simulink model "sim_continuo_vs_discreto_control_integral"  (R2016a)
settings: Solver=VariableStepAuto  StartTime=0.0  StopTime=0.2  RelTol=1e-5
values from neighbouring files (symbols this model uses):
  A = [0 1 ... (first row only)    [calculate_gains.m]    (also in get_linear_model.m = jacobian(xp_nl,x_state))
  B = [0 ... (first row only)    [calculate_gains.m]    (also in get_linear_model.m = jacobian(xp_nl,u_state))
  C = [1 0]    [calculate_gains.m]    (also in get_linear_model.m = jacobian(y_nl,x_state))
  Kdi = calc_discrete_integral_controller_gains(A,B,C,Pi,Ts)    [generate_lookup_table.m]
  Ki = calc_integral_controller_gains(A,B,C,Pi)    [generate_lookup_table.m]
  Ts = 4e-4    (= 0.0004)    [calculate_gains.m]    (also in generate_lookup_table.m = 0.0005)
undefined symbols (not defined in the file or in its folder): Ad, Bd, Cd, DiscIntNeverNeededParam, Kdo, Ko
settings Model: Creator=manuel  LastModifiedBy=manuel

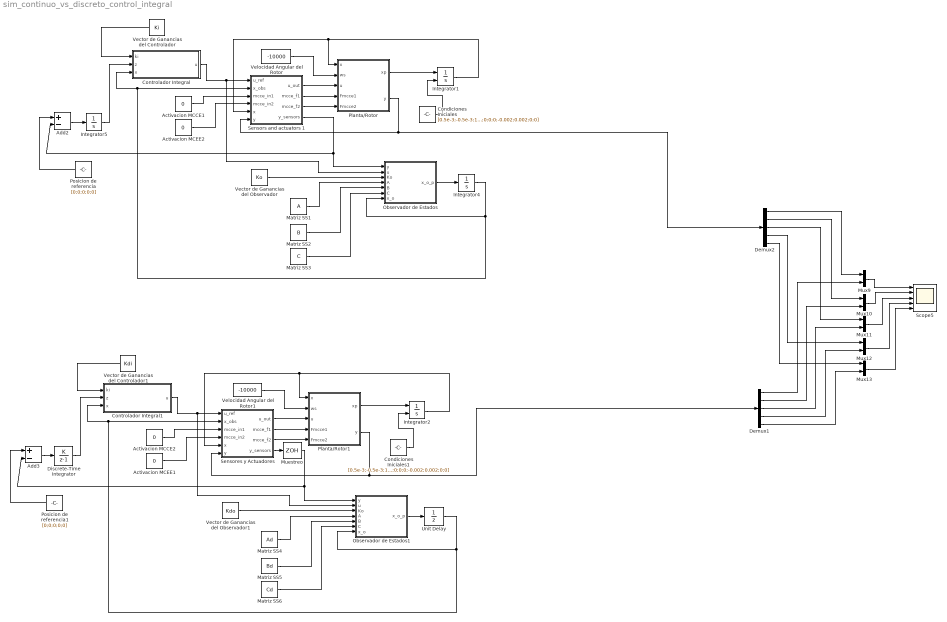
== system sim_continuo_vs_discreto_control_integral ==
  Activacion MCCE1 : Constant  Value=0
  Activacion MCCE2 : Constant  Value=0
  Activacion MCEE1 : Constant  Value=0
  Activacion MCEE2 : Constant  Value=0
  Add2 : Sum  Inputs=+-
  Add3 : Sum  Inputs=+-
  Condiciones Iniciales : Constant  Value=[0.5e-3;-0.5e-3;1e-3;0;0;0;-0.002;0.002;0;0]
  Condiciones Iniciales1 : Constant  Value=[0.5e-3;-0.5e-3;1e-3;0;0;0;-0.002;0.002;0;0]
  Controlador Integral : MATLAB Function  TreatAsAtomicUnit=on
  Controlador Integral1 : MATLAB Function  TreatAsAtomicUnit=on
  Demux1 : Demux  Outputs=5
  Demux2 : Demux  Outputs=5
  Discrete-Time Integrator : DiscreteIntegrator  IntegratorMethod=Accumulation: Forward Euler  gainval=1  InitialCondition=[0;0;0;0;0]  InitialConditionSetting=State (most efficient)  SampleTime=-1  ICPrevOutput=DiscIntNeverNeededParam  ICPrevScaledInput=DiscIntNeverNeededParam
  Integrator1 : Integrator  InitialConditionSource=external  InitialCondition=[0;0;0;0;0;0;0;0;0;0]
  Integrator2 : Integrator  InitialConditionSource=external  InitialCondition=[0;0;0;0;0;0;0;0;0;0]
  Integrator4 : Integrator  InitialCondition=[0;0;0;0;0;0;0;0;0;0]
  Integrator5 : Integrator  InitialCondition=[0;0;0;0;0]
  Matriz SS1 : Constant  Value=A  VectorParams1D=off
  Matriz SS2 : Constant  Value=B  VectorParams1D=off
  Matriz SS3 : Constant  Value=C  VectorParams1D=off
  Matriz SS4 : Constant  Value=Ad  VectorParams1D=off
  Matriz SS5 : Constant  Value=Bd  VectorParams1D=off
  Matriz SS6 : Constant  Value=Cd  VectorParams1D=off
  Muestreo : ZeroOrderHold  SampleTime=Ts
  Mux{9..13} (5 alike) : Mux  Inputs=2
  Observador de Estados : MATLAB Function  TreatAsAtomicUnit=on
  Observador de Estados1 : MATLAB Function  TreatAsAtomicUnit=on
  Planta/Rotor : MATLAB Function  TreatAsAtomicUnit=on
  Planta/Rotor1 : MATLAB Function  TreatAsAtomicUnit=on
  Posicion de referencia : Constant  Value=[0;0;0;0;0]
  Posicion de referencia1 : Constant  Value=[0;0;0;0;0]
  Scope5 : Scope  NumInputPorts=5
  Sensores y Actuadores : Subsystem
  Sensors and actuators 1 : Subsystem
  Unit Delay : UnitDelay  InitialCondition=[0;0;0;0;0;0;0;0;0;0]  SampleTime=-1
  Vector de Ganancias del Controlador : Constant  Value=Ki  VectorParams1D=off
  Vector de Ganancias del Controlador1 : Constant  Value=Kdi  VectorParams1D=off
  Vector de Ganancias del Observador : Constant  Value=Ko  VectorParams1D=off
  Vector de Ganancias del Observador1 : Constant  Value=Kdo  VectorParams1D=off
  Velocidad Angular del Rotor : Constant  Value=-10000  VectorParams1D=off
  Velocidad Angular del Rotor1 : Constant  Value=-10000  VectorParams1D=off
  wires:
  Mux9/1 -> Scope5/1
  Mux10/1 -> Scope5/2
  Mux11/1 -> Scope5/3
  Mux12/1 -> Scope5/4
  Mux13/1 -> Scope5/5
  Demux1/2 -> Mux10/2
  Demux1/1 -> Mux9/2
  Demux1/3 -> Mux11/2
  Demux1/4 -> Mux12/2
  Demux1/5 -> Mux13/2
  Demux2/1 -> Mux9/1
  Demux2/2 -> Mux10/1
  Demux2/3 -> Mux11/1
  Demux2/4 -> Mux12/1
  Demux2/5 -> Mux13/1
  Integrator1/1 -> Planta/Rotor/1(x), Sensors and actuators 1/5(x)
  Add2/1 -> Integrator5/1
  Planta/Rotor/1(xp) -> Integrator1/1
  Observador de Estados/1(x_o_p) -> Integrator4/1
  Vector de Ganancias del Observador/1 -> Observador de Estados/3(Ko)
  Matriz SS1/1 -> Observador de Estados/4(A)
  Matriz SS2/1 -> Observador de Estados/5(B)
  Matriz SS3/1 -> Observador de Estados/6(C)
  Vector de Ganancias del Controlador/1 -> Controlador Integral/1(ki)
  Posicion de referencia/1 -> Add2/1
  Integrator5/1 -> Controlador Integral/2(z)
  Controlador Integral/1(u) -> Observador de Estados/2(u), Sensors and actuators 1/1(u_ref)
  Integrator4/1 -> Sensors and actuators 1/2(x_obs), Controlador Integral/3(x), Observador de Estados/7(x_o)
  Activacion MCCE1/1 -> Sensors and actuators 1/3(mcce_in1)
  Activacion MCEE2/1 -> Sensors and actuators 1/4(mcce_in2)
  Sensors and actuators 1/1(u_out) -> Planta/Rotor/3(u)
  Sensors and actuators 1/2(mcce_f1) -> Planta/Rotor/4(Fmcce1)
  Sensors and actuators 1/3(mcce_f2) -> Planta/Rotor/5(Fmcce2)
  Sensors and actuators 1/4(y_sensors) -> Observador de Estados/1(y), Add2/2
  Condiciones Iniciales/1 -> Integrator1/2
  Velocidad Angular del Rotor/1 -> Planta/Rotor/2(ws)
  Integrator2/1 -> Sensores y Actuadores/5(x), Planta/Rotor1/1(x)
  Planta/Rotor1/1(xp) -> Integrator2/1
  Observador de Estados1/1(x_o_p) -> Unit Delay/1
  Vector de Ganancias del Observador1/1 -> Observador de Estados1/3(Ko)
  Matriz SS4/1 -> Observador de Estados1/4(A)
  Matriz SS5/1 -> Observador de Estados1/5(B)
  Matriz SS6/1 -> Observador de Estados1/6(C)
  Vector de Ganancias del Controlador1/1 -> Controlador Integral1/1(ki)
  Posicion de referencia1/1 -> Add3/1
  Controlador Integral1/1(u) -> Sensores y Actuadores/1(u_ref), Observador de Estados1/2(u)
  Unit Delay/1 -> Observador de Estados1/7(x_o), Controlador Integral1/3(x), Sensores y Actuadores/2(x_obs)
  Activacion MCCE2/1 -> Sensores y Actuadores/3(mcce_in1)
  Activacion MCEE1/1 -> Sensores y Actuadores/4(mcce_in2)
  Sensores y Actuadores/1(u_out) -> Planta/Rotor1/3(u)
  Sensores y Actuadores/2(mcce_f1) -> Planta/Rotor1/4(Fmcce1)
  Sensores y Actuadores/3(mcce_f2) -> Planta/Rotor1/5(Fmcce2)
  Planta/Rotor1/2(y) -> Demux1/1, Sensores y Actuadores/6(y)
  Sensores y Actuadores/4(y_sensors) -> Muestreo/1
  Condiciones Iniciales1/1 -> Integrator2/2
  Velocidad Angular del Rotor1/1 -> Planta/Rotor1/2(ws)
  Muestreo/1 -> Add3/2, Observador de Estados1/1(y)
  Add3/1 -> Discrete-Time Integrator/1
  Discrete-Time Integrator/1 -> Controlador Integral1/2(z)
  Planta/Rotor/2(y) -> Sensors and actuators 1/6(y), Demux2/1

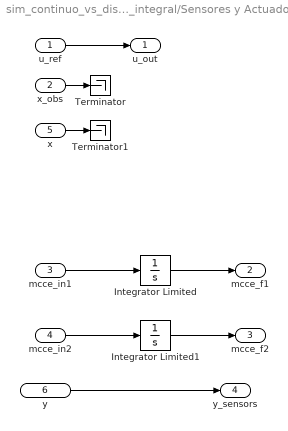
== system sim_continuo_vs_discreto_control_integral/Sensores y Actuadores ==
  u_ref : Inport
  x_obs : Inport  Port=2
  mcce_in1 : Inport  Port=3
  mcce_in2 : Inport  Port=4
  x : Inport  Port=5
  y : Inport  Port=6
  Integrator Limited : Integrator  InitialCondition=6  LimitOutput=on  UpperSaturationLimit=40  LowerSaturationLimit=6
  Integrator Limited1 : Integrator  InitialCondition=6  LimitOutput=on  UpperSaturationLimit=40  LowerSaturationLimit=6
  Terminator : Terminator
  Terminator1 : Terminator
  u_out : Outport
  mcce_f1 : Outport  Port=2
  mcce_f2 : Outport  Port=3
  y_sensors : Outport  Port=4
  wires:
  y/1 -> y_sensors/1
  x/1 -> Terminator1/1
  Integrator Limited1/1 -> mcce_f2/1
  mcce_in2/1 -> Integrator Limited1/1
  mcce_in1/1 -> Integrator Limited/1
  Integrator Limited/1 -> mcce_f1/1
  x_obs/1 -> Terminator/1
  u_ref/1 -> u_out/1

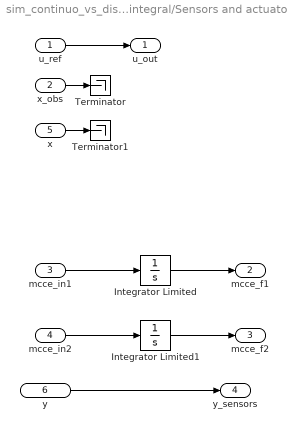
== system sim_continuo_vs_discreto_control_integral/Sensors and actuators 1 ==
  u_ref : Inport
  x_obs : Inport  Port=2
  mcce_in1 : Inport  Port=3
  mcce_in2 : Inport  Port=4
  x : Inport  Port=5
  y : Inport  Port=6
  Integrator Limited : Integrator  InitialCondition=6  LimitOutput=on  UpperSaturationLimit=40  LowerSaturationLimit=6
  Integrator Limited1 : Integrator  InitialCondition=6  LimitOutput=on  UpperSaturationLimit=40  LowerSaturationLimit=6
  Terminator : Terminator
  Terminator1 : Terminator
  u_out : Outport
  mcce_f1 : Outport  Port=2
  mcce_f2 : Outport  Port=3
  y_sensors : Outport  Port=4
  wires:
  u_ref/1 -> u_out/1
  x_obs/1 -> Terminator/1
  Integrator Limited/1 -> mcce_f1/1
  mcce_in1/1 -> Integrator Limited/1
  mcce_in2/1 -> Integrator Limited1/1
  Integrator Limited1/1 -> mcce_f2/1
  x/1 -> Terminator1/1
  y/1 -> y_sensors/1

== matlab function sim_continuo_vs_discreto_control_integral/Controlador Integral ==
  data: ki input; z input; x input; u output
function u  = integral_controller(ki,z,x)
%#codegen
xi = [x;z];
u = -ki*xi;

== matlab function sim_continuo_vs_discreto_control_integral/Observador de Estados ==
  data: y input; u input; x_o_p output; Ko input; A input; B input; C input; x_o input
function x_o_p = state_obsever(y,u,Ko,A,B,C,x_o)
%#codegen
x_o_p = A*x_o + B*u + Ko*(y-C*x_o);

== matlab function sim_continuo_vs_discreto_control_integral/Planta//Rotor ==
  data: xp output; x input; ws input; y output; u input; Fmcce1 input; Fmcce2 input
function [xp,y]  = fcn(x,ws,u,Fmcce1,Fmcce2)
Fd_x = 0;
Fd_y = 0;
Fd_z = 0;
Md_y = 0;
Md_z = 0;
[xp,y] = hmb_non_linear_model(x,u,ws,Fd_x,Fd_y,Fd_z,Md_y,Md_z,Fmcce1,Fmcce2);
end

== matlab function sim_continuo_vs_discreto_control_integral/Controlador Integral1 ==
  data: ki input; z input; x input; u output
function u  = integral_controller(ki,z,x)
%#codegen
xi = [x;z];
u = -ki*xi;

== matlab function sim_continuo_vs_discreto_control_integral/Observador de Estados1 ==
  data: y input; u input; x_o_p output; Ko input; A input; B input; C input; x_o input
function x_o_p = state_obsever(y,u,Ko,A,B,C,x_o)
%#codegen
x_o_p = A*x_o + B*u + Ko*(y-C*x_o);

== matlab function sim_continuo_vs_discreto_control_integral/Planta//Rotor1 ==
  data: xp output; x input; ws input; y output; u input; Fmcce1 input; Fmcce2 input
function [xp,y]  = fcn(x,ws,u,Fmcce1,Fmcce2)
Fd_x = 0;
Fd_y = 0;
Fd_z = 0;
Md_y = 0;
Md_z = 0;
[xp,y] = hmb_non_linear_model(x,u,ws,Fd_x,Fd_y,Fd_z,Md_y,Md_z,Fmcce1,Fmcce2);
end
